simulink model "test"  (R2013b)
settings: Solver=ode45  StartTime=0.0  StopTime=10.0  RelTol=1e-3
settings Model: Creator=qiji  LastModifiedBy=qiji

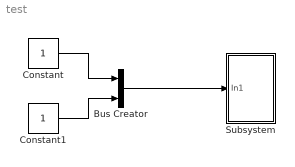
== system test ==
  Bus Creator : BusCreator  Inputs=2
  Constant : Constant
  Constant1 : Constant
  Subsystem : Subsystem
  wires:
  Constant/1 -> Bus Creator/1
  Constant1/1 -> Bus Creator/2
  Bus Creator/1 -> Subsystem/1(In1)

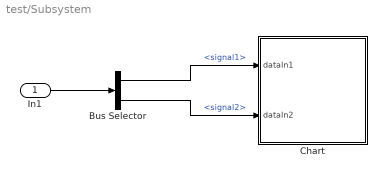
== system test/Subsystem ==
  In1 : Inport  PortDimensions=2
  Bus Selector : BusSelector  OutputSignals=signal1,signal2
  Chart : Stateflow chart  TreatAsAtomicUnit=on
  wires:
  In1/1 -> Bus Selector/1
  Bus Selector/1 -> Chart/1(dataIn1)  "<signal1>"
  Bus Selector/2 -> Chart/2(dataIn2)  "<signal2>"

== stateflow chart test/Subsystem/Chart ==
  state start
  (default) -> start : {
      | dataIn1;
      | dataIn2;
      | }
  data: dataIn1 input double; dataIn2 input double
